simulink model "EKF_Sim_FAEKF"  (R2022b)
settings: Solver=ode4  StartTime=time_start  StopTime=time_end  FixedStep=time_step  MaxStep=0.1  RelTol=1e-6  AbsTol=1e-6
values from neighbouring files (symbols this model uses):
  COE_chaser = [theta0_chaser a_chaser e_chaser                          i_chaser RAAN_chaser AoP_chaser]    [FFNAV_EKF_MakeParams.m]
  COE_target = [theta0_target a_target e_target                          i_target RAAN_target AoP_target]    [FFNAV_EKF_MakeParams.m]
  FUZZY_props = FFNAV_FAEKF_FuzzyInitialize(MSFplot_flag)    [FFNAV_FAEKF_RunSim.m]
  GPS_r_STD = [1.20 1.20 1.20]    [FFNAV_EKF_MakeParams.m]    (also in FFNAV_FAEKF_RunSim.m = 10*GPS_r_STD)
  GPS_v_STD = [0.03 0.03 0.03]    [FFNAV_EKF_MakeParams.m]    (also in FFNAV_FAEKF_RunSim.m = 10*GPS_v_STD)
  mu = Constants.mu_Earth    [FFNAV_EKF_MakeParams.m]    (also in FFNAV_relative_motion_diff_eqns.m)
  N_window = 30    [FFNAV_FAEKF_RunSim.m]
  Q0 = [ sig2_r        0 0 0 0 0 0 0 0 0 ... (first row only)    [FFNAV_EKF_MakeParams.m]    (also in FFNAV_FAEKF_RunSim.m = 10*Q0)
  Q_adapt = Q0    [FFNAV_FAEKF_FuzzyAdapt.m]    (also in FFNAV_FAEKF_RunSim.m = 0)
  R0 = [ sig2_rm     0 0 0 0 0 0 ... (first row only)    [FFNAV_EKF_MakeParams.m]    (also in FFNAV_FAEKF_RunSim.m = R0)
  R_adapt = R0*beta^(-2*(k))    [FFNAV_FAEKF_FuzzyAdapt.m]    (also in FFNAV_FAEKF_RunSim.m = 0)
  theta0_target = 0    [FFNAV_EKF_MakeParams.m]
  time_step = 1    [FFNAV_FAEKF_RunSim.m]
undefined symbols (not defined in the file or in its folder): Constants, n, PropOptions_chaser, PropOptions_target
libraries: dspindex x9, dspstat3 x7, dspmtrx3 x1
(part 2 of 2)

== matlab function EKF_Sim_FAEKF/Kalman Filter/MLE-EKF/MATLAB Function ==
  data: Storage_out output; Storage_in input; state_pre input; sensors input; EKF_out output; Q input; R input; L output; Q_update output; R_update output; time_step parameter; mu parameter; Q_adapt parameter; R_adapt parameter
  function [Storage_out, EKF_out, L, Q_update, R_update] = ...
      USE_EKF_MLE(Storage_in,state_pre,sensors,Q,R,time_step,mu,Q_adapt,R_adapt)
%% USE_EKF ===============================================================
% Description: This function calls the FFNAV_EKF Function, which completes 
% the covariance propagation and correction phases of the EKF algorithm. 
% The output is then passed back to the simulink model.

EKF_out     = zeros(243,1);
Storage_out = zeros(334,1);
Q_update    = zeros(10,10);
R_update    = zeros(7,7);

[EKF_out, Storage_out, L, Q_update, R_update] = ...
    FFNAV_EKF_MLE(Storage_in,time_step,mu,state_pre,sensors,Q,R,Q_adapt,R_adapt);
end
% ========================================================================

== matlab function EKF_Sim_FAEKF/Kalman Filter/FAEKF/Adaptations/Theoretical Covariances ==
  data: Pr_vector input; y output
function y = fcn(Pr_vector)
%#codegen

Pr_theo = [         Pr_vector(1:7)'
                    Pr_vector(8:14)'
                    Pr_vector(15:21)'
                    Pr_vector(22:28)'
                    Pr_vector(29:35)'
                    Pr_vector(36:42)'
                    Pr_vector(43:49)'];
                
Pr_theo_diag = diag(Pr_theo);
   
y = Pr_theo_diag;

== matlab function EKF_Sim_FAEKF/Kalman Filter/FAEKF/Adaptations/USE_FuzzyAdapt ==
  data: state_pre input; Pr_theo input; Pr_smooth input; residuals input; time input; FUZZY_props parameter; Q_pre input; R_pre input; time_step parameter; mu parameter; Q0 parameter; R0 parameter; NIS output; deltaDOD output; DOD_true output; Q output; R output; epsilon_Q output; epsilon_R output; R_adapt parameter; Q_adapt parameter
   function [NIS, deltaDOD, DOD_true, Q,R, epsilon_Q, epsilon_R] = ...
       USE_FuzzyAdapt(state_pre, Pr_theo, Pr_smooth, residuals, ...
     time, FUZZY_props, Q_pre, R_pre, time_step, mu, Q0, R0, R_adapt, Q_adapt)
%% USE_EKF ===============================================================
% ========================================================================
% Description: This block calls the FFNAV_EKF Fuzzy Adaptation function, 
% which calculates an update of the process and measurement noise  
% covariance matrices.

Q = zeros(10,10);
R = zeros(7,7);

[Q, R, NIS, deltaDOD, DOD_true, epsilon_Q, epsilon_R] = ...
    FFNAV_FAEKF_FuzzyAdapt(state_pre, Pr_theo, Pr_smooth, residuals, ...
    time_step, mu, Q0, R0, Q_pre, R_pre, time, FUZZY_props, Q_adapt, R_adapt);

end
% ========================================================================

== matlab function EKF_Sim_FAEKF/Kalman Filter/FAEKF/EKF Correction/MATLAB Function ==
  data: sensors input; input_priori input; output output; R input
 function output = USE_FAEKF_Correction(sensors, input_priori, R)
%% USE_EKF ===============================================================
% ========================================================================
% Description: This function calls the FFNAV_EKF Function, which completes 
% the covariance propagation and correction phases of the EKF algorithm. 
% The output is then passed back to the simulink model.

output = zeros(243,1);
[output] = FFNAV_FAEKF_Correction(input_priori, sensors, R);
end
% ========================================================================

== matlab function EKF_Sim_FAEKF/Kalman Filter/FAEKF/EKF Propagation/MATLAB Function ==
  data: state_pre input; output output; Q input; time_step parameter; mu parameter
 function output = USE_FAEKF_Propagation(state_pre, Q, time_step, mu)
%% USE_EKF ===============================================================
% ========================================================================
% Description: This function calls the FFNAV_EKF Function, which completes 
% the covariance propagation and correction phases of the EKF algorithm. 
% The output is then passed back to the simulink model.

output = zeros(110,1);
output = FFNAV_FAEKF_Propagation(state_pre, time_step, mu, Q);
end
% ========================================================================

== matlab function EKF_Sim_FAEKF/GPS Measurements /Orbital Mechanics for Target Spacecraft/MATLAB Function1 ==
  data: R_Sat input; V_Sat input; r_ddot output; Constants parameter; PropOptions_target parameter
function r_ddot = r_ddot(R_Sat, V_Sat, Constants, PropOptions_target )
% ========================================================================
% Description: This function calculates -mu/r^3 *r to propagate the radius
% vector of the orbital motion

coder.extrinsic('Accelerations');

r_ddot = zeros(3,1);
r_ddot = Accelerations(R_Sat, V_Sat, Constants, PropOptions_target);

end
% ========================================================================

== matlab function EKF_Sim_FAEKF/GPS Measurements /Orbital Mechanics for Target Spacecraft/Target Orbital Mechanics ==
  data: v_ECI output; r_ECI output; mu parameter; COE_target parameter
 function [v_ECI,r_ECI] = Orb_Mech(mu, COE_target)
% ========================================================================
% Description: This funciton calculates the initial r and v vectors, 
% given the provided classiclal orbital elements defined in the
% initialization of the simulation.

%%========================================================================
%Extract COE values
theta       = COE_target(1);
a           = COE_target(2);
e           = COE_target(3);
i           = COE_target(4);
RAAN        = COE_target(5);
w           = COE_target(6);

%%========================================================================
p   = a*(1-e^2);                                                %Defining the semilatus rectum (Eq. 2.31)
r   = p/(1+e*cos(theta));                               %Defining the radius (Eq. 2.32)

r_P = [r*cos(theta) r*sin(theta) 0]';                           %(r in perifocal frame - Eq. 2.86) 
v_P = [-sqrt(mu/p)*sin(theta) sqrt(mu/p)*(e+cos(theta)) 0]';    %(v in perifocal frame - Eq. 2.87)

%Rotation Matrix from P to ECI Frame
C_IP = [    cos(RAAN)*cos(w)-sin(RAAN)*cos(i)*sin(w) -cos(RAAN)*sin(w)-sin(RAAN)*cos(i)*cos(w) sin(RAAN)*sin(i);
            sin(RAAN)*cos(w)+cos(RAAN)*cos(i)*sin(w) -sin(RAAN)*sin(w)+cos(RAAN)*cos(i)*cos(w) -cos(RAAN)*sin(i);
                        sin(i)*sin(w)                            sin(i)*cos(w)                       cos(i)  ];

%Definition of ECI Frame
x_ECI   = [1 0 0];
y_ECI   = [0 1 0];
z_ECI   = [0 0 1];
F_ECI   = [x_ECI; y_ECI; z_ECI]; %Reference Frame ECI

%r and v vectors in ECI Frame
r_ECI   = F_ECI*C_IP*r_P;
v_ECI   = F_ECI*C_IP*v_P;

%z_vec_ECI  = cross(r_ECI, v_ECI)/norm(cross(r_ECI, v_ECI));    %Check orientation of z vector
%X_ECI      = [r_ECI v_ECI]';                                   %State Vector in ECI components (Eq. 2.82)

r_mag = norm(r_ECI);
r_hat = r_ECI/r_mag;

end
% ========================================================================

== matlab function EKF_Sim_FAEKF/GPS Measurements /Orbital Mechanics for Chaser Spacecraft/MATLAB Function1 ==
  data: R_Sat input; r_ddot output; V_Sat input; Constants parameter; PropOptions_chaser parameter
function r_ddot = r_ddot(R_Sat, V_Sat, Constants, PropOptions_chaser)
% ========================================================================
% Description: This function calculates -mu/r^3 *r to propagate the radius
% vector of the orbital motion

coder.extrinsic('Accelerations');

r_ddot = zeros(3,1);
r_ddot = Accelerations(R_Sat, V_Sat, Constants, PropOptions_chaser);

end
% ========================================================================
